simulink model "CurrPowerLimCalc"  (R2024b)
settings: configuration reference "BMS_Sw_CodeGenConfig" (kept outside this file)
undefined symbols (not defined in the file): Battery, OverCellVoltageLimit, ts, UnderCellVoltageLimit
settings Model: DataDictionary=DD_CurrPowerLimCalc.sldd  EnableAccessToBaseWorkspace=off  ExtModeTrigDuration=5  Creator=cpatel  LastModifiedBy=18811
settings ConfigSetRef: SourceName=BMS_Sw_CodeGenConfig

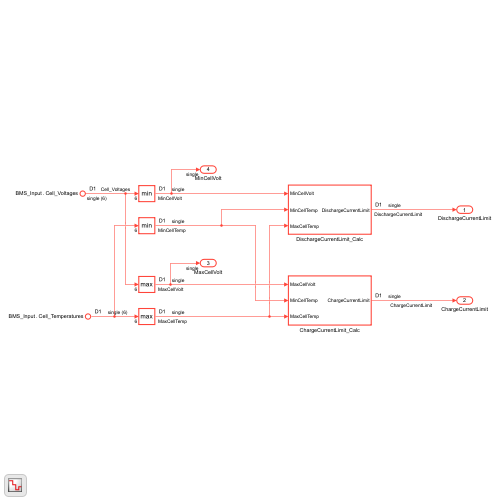
[thumbnail: Simulink's stored preview of the top-level diagram]
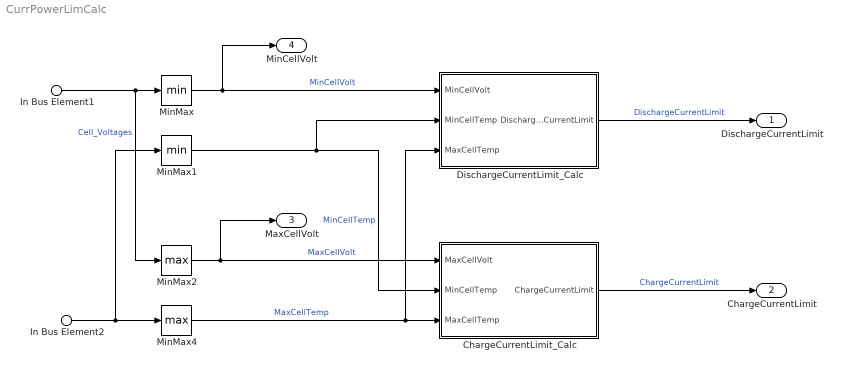
== system CurrPowerLimCalc ==
  In Bus Element1 : Inport  PortName=BMS_Input  Element=Cell_Voltages
  In Bus Element2 : Inport  PortName=BMS_Input  Element=Cell_Temperatures
  ChargeCurrentLimit_Calc : Subsystem
  DischargeCurrentLimit_Calc : Subsystem
  MinMax : MinMax
  MinMax1 : MinMax
  MinMax2 : MinMax  Function=max
  MinMax4 : MinMax  Function=max
  DischargeCurrentLimit : Outport
  ChargeCurrentLimit : Outport  Port=2
  MaxCellVolt : Outport  Port=3  OutDataTypeStr=single  PortDimensions=1  SampleTime=[0.10000000000000001,0]  VectorParamsAs1DForOutWhenUnconnected=off
  MinCellVolt : Outport  Port=4  OutDataTypeStr=single  PortDimensions=1  SampleTime=[0.10000000000000001,0]  VectorParamsAs1DForOutWhenUnconnected=off
  wires:
  ChargeCurrentLimit_Calc/1(ChargeCurrentLimit) -> ChargeCurrentLimit/1  "ChargeCurrentLimit"
  DischargeCurrentLimit_Calc/1(DischargeCurrentLimit) -> DischargeCurrentLimit/1  "DischargeCurrentLimit"
  In Bus Element1/1 -> MinMax2/1, MinMax/1  "Cell_Voltages"
  In Bus Element2/1 -> MinMax4/1, MinMax1/1
  MinMax2/1 -> ChargeCurrentLimit_Calc/1(MaxCellVolt), MaxCellVolt/1  "MaxCellVolt"
  MinMax/1 -> DischargeCurrentLimit_Calc/1(MinCellVolt), MinCellVolt/1  "MinCellVolt"
  MinMax4/1 -> DischargeCurrentLimit_Calc/3(MaxCellTemp), ChargeCurrentLimit_Calc/3(MaxCellTemp)  "MaxCellTemp"
  MinMax1/1 -> DischargeCurrentLimit_Calc/2(MinCellTemp), ChargeCurrentLimit_Calc/2(MinCellTemp)  "MinCellTemp"

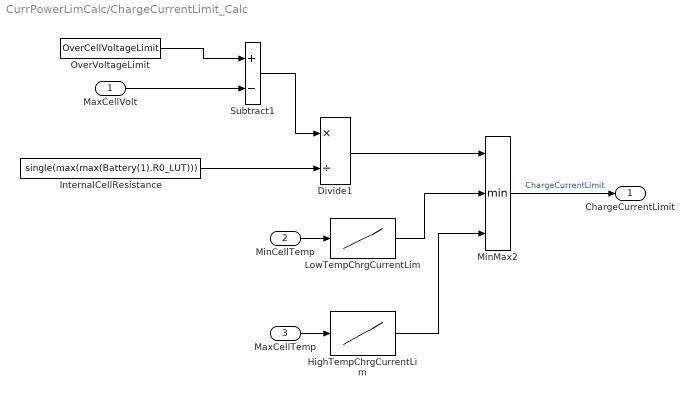
== system CurrPowerLimCalc/ChargeCurrentLimit_Calc ==
  MaxCellVolt : Inport
  MinCellTemp : Inport  Port=2
  MaxCellTemp : Inport  Port=3
  Divide1 : Product  Inputs=*/
  HighTempChrgCurrentLim : Lookup_n-D  NumberOfTableDimensions=1  BreakpointsForDimension1=273.15+[-30:1:70]  Table=50*(1-tanh(273.15+[-30:1:70]-273.15-50))/2  InternalRulePriority=Speed  RndMeth=Simplest
  InternalCellResistance : Constant  Value=single(max(max(Battery(1).R0_LUT)))  OutDataTypeStr=single  SampleTime=ts
  LowTempChrgCurrentLim : Lookup_n-D  NumberOfTableDimensions=1  BreakpointsForDimension1=273.15+[-30:1:70]  Table=50*(1+tanh(273.15+[-30:1:70]-(273.15)))/2  InternalRulePriority=Speed  RndMeth=Simplest
  MinMax2 : MinMax  Inputs=3
  OverVoltageLimit : Constant  Value=OverCellVoltageLimit  OutDataTypeStr=single  SampleTime=ts
  Subtract1 : Sum  Inputs=+-
  ChargeCurrentLimit : Outport  VectorParamsAs1DForOutWhenUnconnected=off
  wires:
  OverVoltageLimit/1 -> Subtract1/1
  MinMax2/1 -> ChargeCurrentLimit/1  "ChargeCurrentLimit"
  MaxCellVolt/1 -> Subtract1/2
  Subtract1/1 -> Divide1/1
  Divide1/1 -> MinMax2/1
  InternalCellResistance/1 -> Divide1/2
  MinCellTemp/1 -> LowTempChrgCurrentLim/1
  MaxCellTemp/1 -> HighTempChrgCurrentLim/1
  HighTempChrgCurrentLim/1 -> MinMax2/3
  LowTempChrgCurrentLim/1 -> MinMax2/2

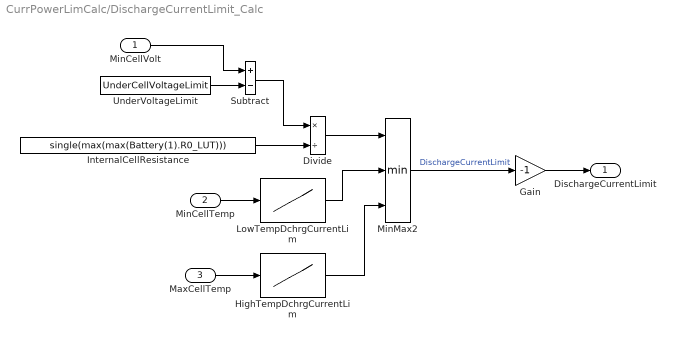
== system CurrPowerLimCalc/DischargeCurrentLimit_Calc ==
  MinCellVolt : Inport
  MinCellTemp : Inport  Port=2
  MaxCellTemp : Inport  Port=3
  Divide : Product  Inputs=*/
  Gain : Gain  Gain=-1
  HighTempDchrgCurrentLim : Lookup_n-D  NumberOfTableDimensions=1  BreakpointsForDimension1=273.15+[-30:1:70]  Table=100*(1-tanh(273.15+[-30:1:70]-273.15-50))/2  InternalRulePriority=Speed  RndMeth=Simplest
  InternalCellResistance : Constant  Value=single(max(max(Battery(1).R0_LUT)))  OutDataTypeStr=single  SampleTime=ts
  LowTempDchrgCurrentLim : Lookup_n-D  NumberOfTableDimensions=1  BreakpointsForDimension1=273.15+[-30:1:70]  Table=100*(1+tanh(273.15+[-30:1:70]-(273.15)))/2  InternalRulePriority=Speed  RndMeth=Simplest
  MinMax2 : MinMax  Inputs=3
  Subtract : Sum  Inputs=+-
  UnderVoltageLimit : Constant  Value=UnderCellVoltageLimit  OutDataTypeStr=single  SampleTime=ts
  DischargeCurrentLimit : Outport  VectorParamsAs1DForOutWhenUnconnected=off
  wires:
  MinMax2/1 -> Gain/1  "DischargeCurrentLimit"
  Divide/1 -> MinMax2/1
  MinCellVolt/1 -> Subtract/1
  InternalCellResistance/1 -> Divide/2
  Subtract/1 -> Divide/1
  UnderVoltageLimit/1 -> Subtract/2
  Gain/1 -> DischargeCurrentLimit/1
  MaxCellTemp/1 -> HighTempDchrgCurrentLim/1
  MinCellTemp/1 -> LowTempDchrgCurrentLim/1
  HighTempDchrgCurrentLim/1 -> MinMax2/3
  LowTempDchrgCurrentLim/1 -> MinMax2/2
